simulink subsystem "VOO_mode"  (R2022a)
settings: Solver=VariableStepAuto  StartTime=0.0  StopTime=10.0  RelTol=1e-3
settings Model: Creator=ivanl  LastModifiedBy=ivanl

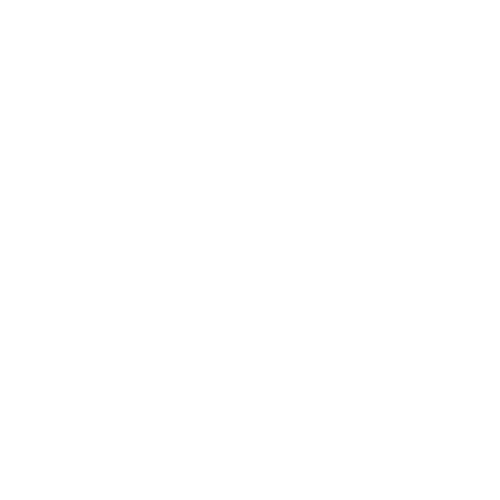
[thumbnail: Simulink's stored preview of the top-level diagram]
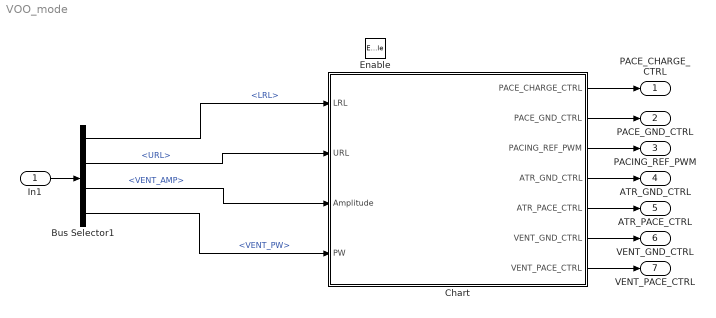
== system VOO_mode ==
  In1 : Inport
  Enable : EnablePort
  Bus Selector1 : BusSelector  OutputSignals=LRL,URL,VENT_AMP,VENT_PW
  Chart : Stateflow chart  TreatAsAtomicUnit=on
      settings: PortSchema="{\"entries\":[{\"content\":{\"sides\":[{\"content\":{\"connectorIds\":[\"In2\",\"In1\",\"In3\",\"In4\"]},\"type\":\"ConnectorPlacement.EquallySpacedRectSide\",\"uuid\":\"608193ca-bbb1-478b-9889-7801dfa3b18f\"},{\"content\":{\"connectorIds\":[\"Out1\",\"Out2\",\"Out3\",\"Out4\",\"Out5\",\"Out6\",\"Out7\"],\"side\":\"RIGHT\"},\"type\":\"ConnectorPlacement.EquallySpacedRectSide\",\"uuid\":\"1c44b789-26b9-4f10-95e3-91179da0d016\"},{\"content\":{\"connectorIds\":[],\"side\":\"TOP\"},\"type\":\"ConnectorPlacement.EquallySpacedRectSide\",\"uuid\":\"49a6d3e9-6382-40aa-95f2-9d63b6dd6751\"}]},\"type\":\"ConnectorPlacement.EquallySpacedConnector\",\"uuid\":\"4b48ab96-7c59-405b-8c63-39a4663f1d1f\"}],\"packageUris\":[\"http://schema.mathworks.com/mf0/Connector/R2020b\"],\"version\":\"1.0\"}"
  PACE_CHARGE_CTRL : Outport
  PACE_GND_CTRL : Outport  Port=2
  PACING_REF_PWM : Outport  Port=3
  ATR_GND_CTRL : Outport  Port=4
  ATR_PACE_CTRL : Outport  Port=5
  VENT_GND_CTRL : Outport  Port=6
  VENT_PACE_CTRL : Outport  Port=7
  wires:
  Chart/7(VENT_PACE_CTRL) -> VENT_PACE_CTRL/1
  Chart/6(VENT_GND_CTRL) -> VENT_GND_CTRL/1
  Chart/5(ATR_PACE_CTRL) -> ATR_PACE_CTRL/1
  Chart/4(ATR_GND_CTRL) -> ATR_GND_CTRL/1
  Chart/3(PACING_REF_PWM) -> PACING_REF_PWM/1
  Chart/2(PACE_GND_CTRL) -> PACE_GND_CTRL/1
  Chart/1(PACE_CHARGE_CTRL) -> PACE_CHARGE_CTRL/1
  Bus Selector1/1 -> Chart/2(LRL)  "<LRL>"
  Bus Selector1/4 -> Chart/4(PW)  "<VENT_PW>"
  Bus Selector1/3 -> Chart/3(Amplitude)  "<VENT_AMP>"
  Bus Selector1/2 -> Chart/1(URL)  "<URL>"
  In1/1 -> Bus Selector1/1

== stateflow chart VOO_mode/Chart ==
  state C22_CHARGE
    entry:
    ATR_PACE_CTRL = false;
    VENT_PACE_CTRL = false;
    PACING_REF_PWM = (Amplitude / 5) *100;
    PACE_CHARGE_CTRL = true;
    PACE_GND_CTRL = true;
    ATR_GND_CTRL = false;
    VENT_GND_CTRL = true ;
  state C22_DISCHARGE
    entry:
    PACE_CHARGE_CTRL = false;
    PACE_GND_CTRL = true;
    ATR_PACE_CTRL = false;
    ATR_GND_CTRL = false;
    VENT_GND_CTRL = false;
    VENT_PACE_CTRL = true;
  (default) -> C22_CHARGE
  C22_DISCHARGE -> C22_CHARGE : after(PW,msec)
  C22_CHARGE -> C22_DISCHARGE : after(((60000/LRL)-PW),msec)
  data: URL input; LRL input double; Amplitude input double; PW input double; PACE_CHARGE_CTRL output boolean; PACE_GND_CTRL output boolean; PACING_REF_PWM output double; ATR_GND_CTRL output boolean; ATR_PACE_CTRL output boolean; VENT_GND_CTRL output boolean; VENT_PACE_CTRL output boolean
